simulink subsystem "median8"  (R2021b)
settings: Solver=VariableStepAuto  StartTime=0.0  StopTime=10.0  RelTol=1e-3
settings Model: Creator=dileepan  LastModifiedBy=dileepan

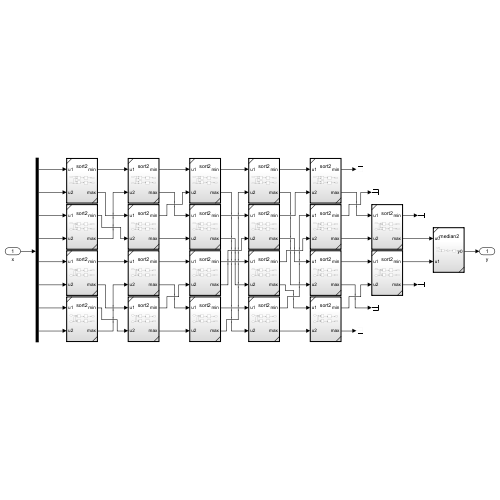
[thumbnail: Simulink's stored preview of the top-level diagram]
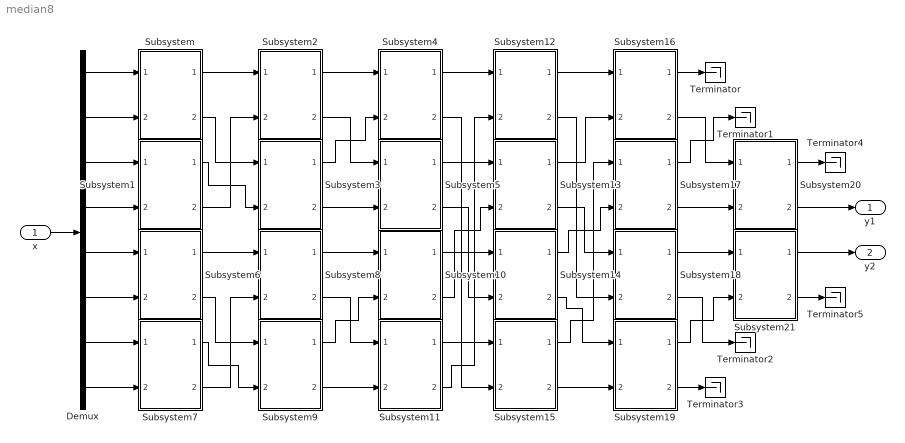
== system median8 ==
  x : Inport
  Demux : Demux  Outputs=8
  Subsystem{,1..21} (22 alike) : Subsystem  TreatAsAtomicUnit=on  ReferencedSubsystem=sort2
  Terminator{,1..5} (6 alike) : Terminator
  y1 : Outport
  y2 : Outport  Port=2
  wires:
  x/1 -> Demux/1
  Demux/1 -> Subsystem/1
  Demux/2 -> Subsystem/2
  Demux/3 -> Subsystem1/1
  Demux/4 -> Subsystem1/2
  Demux/7 -> Subsystem7/1
  Demux/8 -> Subsystem7/2
  Demux/5 -> Subsystem6/1
  Demux/6 -> Subsystem6/2
  Subsystem2/1 -> Subsystem4/1
  Subsystem3/2 -> Subsystem5/2
  Subsystem/1 -> Subsystem2/1
  Subsystem1/2 -> Subsystem2/2
  Subsystem/2 -> Subsystem3/1
  Subsystem1/1 -> Subsystem3/2
  Subsystem8/1 -> Subsystem10/1
  Subsystem9/2 -> Subsystem11/2
  Subsystem8/2 -> Subsystem11/1
  Subsystem9/1 -> Subsystem10/2
  Subsystem2/2 -> Subsystem5/1
  Subsystem3/1 -> Subsystem4/2
  Subsystem6/1 -> Subsystem8/1
  Subsystem7/2 -> Subsystem8/2
  Subsystem6/2 -> Subsystem9/1
  Subsystem7/1 -> Subsystem9/2
  Subsystem16/1 -> Terminator/1
  Subsystem17/2 -> Subsystem20/2
  Subsystem16/2 -> Subsystem20/1
  Subsystem17/1 -> Terminator1/1
  Subsystem18/1 -> Subsystem21/1
  Subsystem18/2 -> Terminator2/1
  Subsystem19/1 -> Subsystem21/2
  Subsystem19/2 -> Terminator3/1
  Subsystem4/1 -> Subsystem12/1
  Subsystem11/1 -> Subsystem15/1
  Subsystem5/1 -> Subsystem13/1
  Subsystem10/1 -> Subsystem14/1
  Subsystem5/2 -> Subsystem14/2
  Subsystem10/2 -> Subsystem13/2
  Subsystem4/2 -> Subsystem15/2
  Subsystem11/2 -> Subsystem12/2
  Subsystem12/1 -> Subsystem16/1
  Subsystem13/1 -> Subsystem16/2
  Subsystem15/2 -> Subsystem19/2
  Subsystem13/2 -> Subsystem18/1
  Subsystem14/1 -> Subsystem17/2
  Subsystem15/1 -> Subsystem17/1
  Subsystem12/2 -> Subsystem18/2
  Subsystem20/1 -> Terminator4/1
  Subsystem21/2 -> Terminator5/1
  Subsystem14/2 -> Subsystem19/1
  Subsystem20/2 -> y1/1
  Subsystem21/1 -> y2/1
